simulink model "solar_PV"  (R2025a)
settings: Solver=ode23t  StartTime=0.0  StopTime=0.2  RelTol=1e-3
undefined symbols (not defined in the file or in its folder): Acid, Lead
libraries: spsSeriesRLCBranchLib x3, spsBatteryLib x1, spsDiodeLib x1, spsMosfetLib x1, spsPVArrayLib x1, simulink x1, sps_lib x1
settings Model: Creator=LENOVO  LastModifiedBy=LENOVO

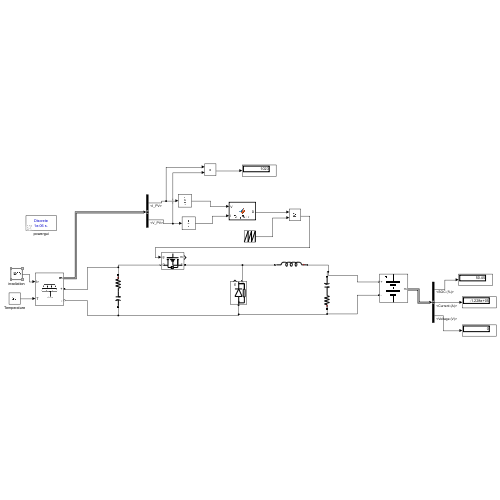
[thumbnail: Simulink's stored preview of the top-level diagram]
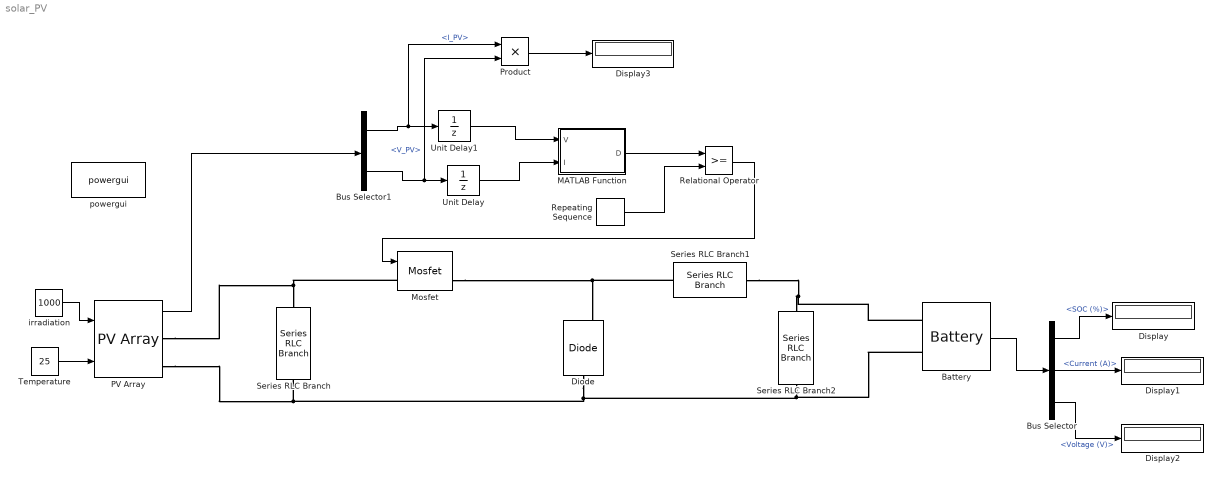
== system solar_PV ==
  Battery : spsBatteryLib/Battery  BatType=Lead-Acid  NomV=12  NomQ=100  SOC=45  Batt_Tr=1  PresetModel=on  MaxQ=104.1667  MinV=9  FullV=13.0658  Dis_rate=20  R=0.0012  Normal_OP=31.0278  expZone="[12.2171     0.333333]"
  Bus Selector : BusSelector  OutputSignals=SOC (%),Current (A),Voltage (V)
  Bus Selector1 : BusSelector  OutputSignals=I_PV,V_PV
  Diode : spsDiodeLib/Diode  Ron=0.001  Lon=0  Vf=0.8  IC=0  UseSnubber=0  Rs=500  Cs=250e-9  Measurements=on
  Display{,1..3} (4 alike) : Display
  MATLAB Function : MATLAB Function  TreatAsAtomicUnit=on
  Mosfet : spsMosfetLib/Mosfet  Ron=0.1  Lon=0  Rd=0.01  Vfd=0  IC=0  Rs=1e5  Cs=inf  Measurements=on
  PV Array : spsPVArrayLib/PV Array  Npar=1  Nser=1  PlotType=array @ 25 deg.C & specified irradiances  S_vec="[ 1000  500  100 ]"  Temp_C_vec="[ 45 25  ]"  ModuleName=A10Green Technology A10J-S72-175  PlotWhenSelected=off  Pm=175.0914  Ncell=72  Voc=43.99  Isc=5.17  Vm=36.63  Im=4.78  beta_Voc_pc=-0.3616  alpha_Isc_pc=0.041509  beta_Voc=-0.15907  alpha_Isc=0.002146  IL=5.178  I0=1.7842e-10  nI=0.98852  Rsh=249.6758  Rs=0.38412  RobustModel=off  RobustCellTemperature=313.3991  BAL=on  Tc=1e-6  Tfilter=5e-5
  Product : Product
  Relational Operator : RelationalOperator  OutDataTypeStr=boolean  RndMeth=Simplest  InputSameDT=off
  Repeating Sequence : simulink/Sources/Repeating Sequence  rep_seq_t=[0 0.002]  rep_seq_y=[0 1]
  Series RLC Branch : spsSeriesRLCBranchLib/Series RLC Branch  LConnTagsString=__new0  RConnTagsString=__new0  BranchType=RC  Resistance=0.0001  Inductance=1e-3  SetiL0=off  InitialCurrent=0  Capacitance=1000e-6  Setx0=on  InitialVoltage=0  Measurements=None
  Series RLC Branch1 : spsSeriesRLCBranchLib/Series RLC Branch  LConnTagsString=__new0  RConnTagsString=__new0  BranchType=L  Resistance=0.0001  Inductance=0.783e-3  SetiL0=off  InitialCurrent=0  Capacitance=1000e-6  Setx0=on  InitialVoltage=0  Measurements=None
  Series RLC Branch2 : spsSeriesRLCBranchLib/Series RLC Branch  LConnTagsString=__new0  RConnTagsString=__new0  BranchType=RC  Resistance=0.0001  Inductance=0.783e-3  SetiL0=off  InitialCurrent=0  Capacitance=364e-6  Setx0=on  InitialVoltage=0  Measurements=None
  Temperature : Constant  Value=25
  Unit Delay : UnitDelay  SampleTime=10e-4  HasFrameUpgradeWarning=on
  Unit Delay1 : UnitDelay  SampleTime=10e-4  HasFrameUpgradeWarning=on
  irradiation : Constant  Value=1000
  powergui : sps_lib/powergui  Priority=1  SimulationMode=Discrete  SampleTime=1e-6  frequency=60  Iterations=50  frequencyindice=0  Pbase=100e6  ErrMax=1e-4  UnitsV=kV  UnitsW=MW  buscounter=0  FunctionMessages=off  echomessages=off  EnableUseOfTLC=off  CurrentSourceSwitches=off  DisableSnubberDevices=off  DisableRonSwitches=off  DisableVfSwitches=off  DisplayEquations=off  AutomaticDiscreteSolvers=off  SolverType=Tustin/Backward Euler (TBE)  Interpol=off  ExternalGateDelay=off  methode=off  Ts=100  x0status=blocks  SPID=on  SwTol=0  HookPort=off  NonlinearTolerance=1e-4  nMaxIteration=100  ContinueOnMaxIteration=off  RestoreLinks=warning  ResistiveCurrentMeasurement=off  Frange=[0:2:500]  Ylog=off  Xlog=on  ShowGrid=off  save=off  variable=ZData  structure=0  ZoomFFT=off  StartTime=0.0  cycles=1  DisplayStyle=1  fundamental=60  FreqAxis=off  MaxFrequency=1000  frequencyindicesteady=1  RmsSteady=1  display=off
  wires:
  irradiation/1 -> PV Array/1
  Temperature/1 -> PV Array/2
  Battery/1 -> Bus Selector/1
  Bus Selector/1 -> Display/1  "<SOC (%)>"
  Bus Selector/2 -> Display1/1  "<Current (A)>"
  Bus Selector/3 -> Display2/1  "<Voltage (V)>"
  PV Array/1 -> Bus Selector1/1
  Bus Selector1/1 -> Product/1, Unit Delay1/1  "<I_PV>"
  Bus Selector1/2 -> Product/2, Unit Delay/1  "<V_PV>"
  Unit Delay1/1 -> MATLAB Function/1(V)
  Unit Delay/1 -> MATLAB Function/2(I)
  Repeating Sequence/1 -> Relational Operator/2
  MATLAB Function/1(D) -> Relational Operator/1
  Relational Operator/1 -> Mosfet/1
  Product/1 -> Display3/1
  connections:
  PV Array/RConn1 -- Series RLC Branch/LConn1 -- Mosfet/LConn1
  PV Array/RConn2 -- Battery/LConn2 -- Series RLC Branch2/LConn1 -- Diode/LConn1 -- Series RLC Branch/RConn1
  Mosfet/RConn1 -- Series RLC Branch1/RConn1 -- Diode/RConn1
  Series RLC Branch1/LConn1 -- Battery/LConn1 -- Series RLC Branch2/RConn1

== matlab function solar_PV/MATLAB Function ==
  data: V input; D output; I input
function D = DutyRatio(V, I)

    Dmax = 0.95;
    Dmin = 0;
    Dinit = 0.95;
    deltaD = 0.0001;
    persistent Vold Pold Dold;

    dataType = 'double';

    if isempty(Vold)
        Vold = 0;
        Pold = 0;
        Dold = Dinit;
    end

    P = V * I;
    dV = V - Vold;
    dP = P - Pold;

    if dP ~= 0
        if dP < 0
            if dV < 0
                D = Dold - deltaD;
            else
                D = Dold + deltaD;
            end
        else
            if dV < 0
                D = Dold + deltaD;
            else
                D = Dold - deltaD;
            end
        end
    else
        D = Dold;
    end

    if D >= Dmax || D <= Dmin
        D = Dold;
    end

    Dold = D;
    Vold = V;
    Pold = P;
end
